simulink model "qam"  (R2021b)
settings: Solver=VariableStepAuto  StartTime=0.0  StopTime=1  RelTol=1e-3
libraries: dspsrcs4 x4, dspfdesign x2
settings Model: Creator=tzajdel  LastModifiedBy=tzajdel

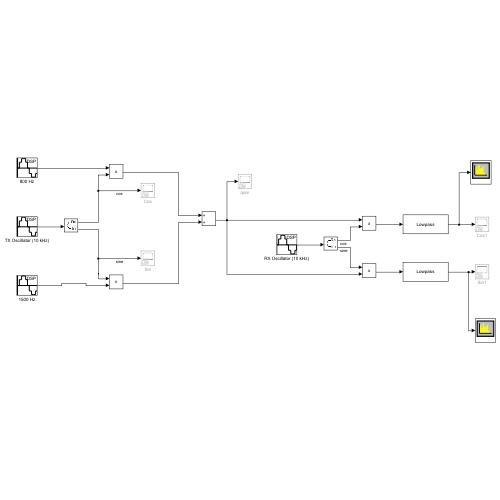
[thumbnail: Simulink's stored preview of the top-level diagram]
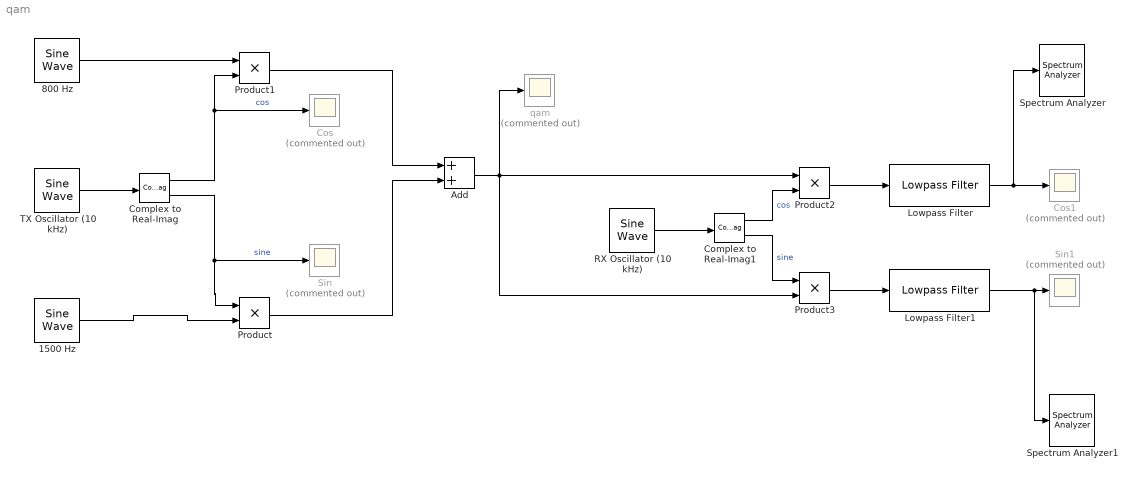
== system qam ==
  1500 Hz : dspsrcs4/Sine Wave  Amplitude=1  Frequency=1500  Phase=0  SampleMode=Discrete  OutComplex=Complex  CompMethod=Trigonometric fcn  TableSize=Speed  SampleTime=1e-5  SamplesPerFrame=100  ResetState=Restart at time zero  OutputFrames=off  dataType=double  wordLen=16  udDataType=sfix(16)  fracBitsMode=Best precision  numFracBits=15  OutDataTypeStr=double  LastOutDataTypeStr=double
  800 Hz : dspsrcs4/Sine Wave  Amplitude=1  Frequency=800  Phase=0  SampleMode=Discrete  OutComplex=Complex  CompMethod=Trigonometric fcn  TableSize=Speed  SampleTime=1e-5  SamplesPerFrame=100  ResetState=Restart at time zero  OutputFrames=off  dataType=double  wordLen=16  udDataType=sfix(16)  fracBitsMode=Best precision  numFracBits=15  OutDataTypeStr=double  LastOutDataTypeStr=double
  Add : Sum
  Complex to Real-Imag : ComplexToRealImag
  Complex to Real-Imag1 : ComplexToRealImag
  Cos : Scope  Commented=on
  Cos1 : Scope  Commented=on
  Lowpass Filter : dspfdesign/Lowpass Filter  FilterType=FIR  DesignForMinimumOrder=on  FilterOrder=50  PassbandFrequency=2e3  StopbandFrequency=3e3  PassbandRipple=0.1  StopbandAttenuation=60  InheritSampleRate=on  SampleRate=44100  SimulateUsing=Interpreted execution  roundingMode=Floor  coeffsDataTypeStr=fixdt(1,16)
  Lowpass Filter1 : dspfdesign/Lowpass Filter  FilterType=FIR  DesignForMinimumOrder=on  FilterOrder=50  PassbandFrequency=2e3  StopbandFrequency=3e3  PassbandRipple=0.1  StopbandAttenuation=60  InheritSampleRate=on  SampleRate=44100  SimulateUsing=Interpreted execution  roundingMode=Floor  coeffsDataTypeStr=fixdt(1,16)
  Product{,1..3} (4 alike) : Product
  RX Oscillator (10 kHz) : dspsrcs4/Sine Wave  Amplitude=1  Frequency=10e3  Phase=0  SampleMode=Discrete  OutComplex=Complex  CompMethod=Trigonometric fcn  TableSize=Speed  SampleTime=1e-5  SamplesPerFrame=100  ResetState=Restart at time zero  OutputFrames=off  dataType=double  wordLen=16  udDataType=sfix(16)  fracBitsMode=Best precision  numFracBits=15  OutDataTypeStr=double  LastOutDataTypeStr=double
  Sin : Scope  Commented=on
  Sin1 : Scope  Commented=on
  Spectrum Analyzer : SpectrumAnalyzer
  Spectrum Analyzer1 : SpectrumAnalyzer
  TX Oscillator (10 kHz) : dspsrcs4/Sine Wave  Amplitude=1  Frequency=10e3  Phase=0  SampleMode=Discrete  OutComplex=Complex  CompMethod=Trigonometric fcn  TableSize=Speed  SampleTime=1e-5  SamplesPerFrame=100  ResetState=Restart at time zero  OutputFrames=off  dataType=double  wordLen=16  udDataType=sfix(16)  fracBitsMode=Best precision  numFracBits=15  OutDataTypeStr=double  LastOutDataTypeStr=double
  qam : Scope  Commented=on
  wires:
  TX Oscillator (10 kHz)/1 -> Complex to Real-Imag/1
  Complex to Real-Imag/1 -> Product1/2, Cos/1  "cos"
  Complex to Real-Imag/2 -> Product/1, Sin/1  "sine"
  800 Hz/1 -> Product1/1
  1500 Hz/1 -> Product/2
  Product1/1 -> Add/1
  Product/1 -> Add/2
  Add/1 -> Product3/2, Product2/1, qam/1
  RX Oscillator (10 kHz)/1 -> Complex to Real-Imag1/1
  Complex to Real-Imag1/1 -> Product2/2  "cos"
  Complex to Real-Imag1/2 -> Product3/1  "sine"
  Product2/1 -> Lowpass Filter/1
  Lowpass Filter/1 -> Spectrum Analyzer/1, Cos1/1
  Product3/1 -> Lowpass Filter1/1
  Lowpass Filter1/1 -> Spectrum Analyzer1/1, Sin1/1
